simulink model "pi_isled"  (R2019b)
settings: Solver=VariableStepAuto  StartTime=0.0  StopTime=t_final  MaxStep=0.001  RelTol=1e-3
values from neighbouring files (symbols this model uses):
  K1 = 1 + 0.1*(2*rand()-1)    [PI_regul.m]
  K2 = 1 + 0.1*(2*rand()-1)    [PI_regul.m]
  Ki = Kia*T0    [PI_regul.m]
  Kia = 1/(2*Tu*Kob)    [PI_regul.m]
  Kp = Kpa    [PI_regul.m]
  Kpa = T1/(2*Tu*Kob)    [PI_regul.m]
  st = 0    [PI_regul.m]
  T0 = 0.1    [PI_regul.m]
  T1 = 1 + 0.1*(2*rand()-1)    [PI_regul.m]
  T2 = 0.8 + 0.1*(2*rand()-1)    [PI_regul.m]
settings Model: Creator=Anton Mayorov  LastModifiedBy=bedla
settings DataIOCC: ReturnWorkspaceOutputs=off
settings DebuggingCC: ArithmeticOperatorsInVariantConditions=warning
settings SFSimCC: SimUseLocalCustomCode=off  CustomCodeUndefinedFunction=UseInterfaceOnly
settings RTWCC: RTWUseLocalCustomCode=off

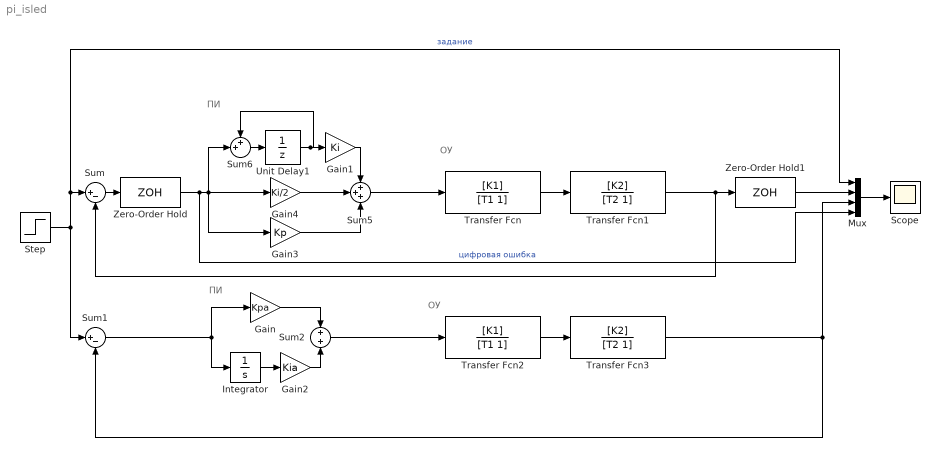
== system pi_isled ==
  note: ПИ
  note: ОУ
  note: ПИ
  note: ОУ
  Gain : Gain  Gain=Kpa
  Gain1 : Gain  Gain=Ki
  Gain2 : Gain  Gain=Kia
  Gain3 : Gain  Gain=Kp
  Gain4 : Gain  Gain=Ki/2
  Integrator : Integrator
  Mux : Mux
  Scope : Scope
  Step : Step  Time=st  SampleTime=0
  Sum : Sum  Inputs=|+-
  Sum1 : Sum  Inputs=|+-
  Sum2 : Sum
  Sum5 : Sum  Inputs=+++
  Sum6 : Sum  Inputs=++|
  Transfer Fcn : TransferFcn  Numerator=[K1]  Denominator=[T1 1]
  Transfer Fcn1 : TransferFcn  Numerator=[K2]  Denominator=[T2 1]
  Transfer Fcn2 : TransferFcn  Numerator=[K1]  Denominator=[T1 1]
  Transfer Fcn3 : TransferFcn  Numerator=[K2]  Denominator=[T2 1]
  Unit Delay1 : UnitDelay  SampleTime=-1  HasFrameUpgradeWarning=on
  Zero-Order Hold : ZeroOrderHold  SampleTime=T0
  Zero-Order Hold1 : ZeroOrderHold  SampleTime=T0
  wires:
  Gain/1 -> Sum2/1
  Transfer Fcn/1 -> Transfer Fcn1/1
  Step/1 -> Mux/1, Sum/1, Sum1/1  "задание"
  Gain2/1 -> Sum2/2
  Integrator/1 -> Gain2/1
  Transfer Fcn1/1 -> Sum/2, Zero-Order Hold1/1
  Zero-Order Hold1/1 -> Mux/2
  Gain3/1 -> Sum5/3
  Unit Delay1/1 -> Sum6/1, Gain1/1
  Mux/1 -> Scope/1
  Gain1/1 -> Sum5/1
  Sum1/1 -> Gain/1, Integrator/1
  Sum2/1 -> Transfer Fcn2/1
  Sum/1 -> Zero-Order Hold/1
  Gain4/1 -> Sum5/2
  Transfer Fcn3/1 -> Sum1/2, Mux/3
  Sum5/1 -> Transfer Fcn/1
  Zero-Order Hold/1 -> Gain4/1, Gain3/1, Sum6/2, Mux/4  "цифровая ошибка"
  Sum6/1 -> Unit Delay1/1
  Transfer Fcn2/1 -> Transfer Fcn3/1
